simulink model "PSM_Commander_ATI"  (R2016a)
settings: Solver=ode3  StartTime=0.0  StopTime=inf  FixedStep=dt  RelTol=1e-3
InitFcn:
  | PSMCMD_DEPENDENCY
  | init_psm_cmd
  | init_scopes
  | init_udp
  | init_resolved_rates
  | ATI_Init_gamma
undefined symbols (not defined in the file or in its folder): A, ATI_torque_convert_to_Nmm, dt, epsilon_vec, f_bias, filter_coeffs_ATI, filter_coeffs_ATI_bias, H_organ2robot, H_robot2organ, inv_T, K_adm, N_ATI, N_ATI_bias, R_organ2robot, R_robot2organ, Rft2organ, scale_vec, v_limits
libraries: slrtlib x5, simulink x4, dspswit3 x4, xpcobsoletelib x3, xpcrtudplib x2, dspsigops x1
settings Model: Creator=Andrea  LastModifiedBy=Long
settings SolverCC: EnableConcurrentExecution=on
settings DataIOCC: LimitDataPoints=on  SaveFormat=Array  SignalLoggingSaveFormat=ModelDataLogs
settings OptimizationCC: BlockReduction=off  OptimizeBlockIOStorage=off  BufferReuse=off  GlobalBufferReuse=off  ExpressionFolding=off  ExpressionDepthLimit=2147483647  LocalBlockOutputs=off  OptimizeModelRefInitCode=on
settings DebuggingCC: UnderspecifiedInitializationDetection=Classic  MergeDetectMultiDrivingBlocksExec=none  SolverPrmCheckMsg=warning  MultiTaskCondExecSysMsg=warning  MultiTaskRateTransMsg=warning  FcnCallInpInsideContextMsg=UseLocalSettings  StateNameClashWarn=warning
settings HardwareCC: ProdBitPerPointer=32  ProdLargestAtomicFloat=None  ProdWordSize=32  ProdLongLongMode=on  ProdHWDeviceType=Generic->32-bit x86 compatible
settings ModelReferenceCC: PropagateSignalLabelsOutOfModel=off
settings SFSimCC: SimParseCustomCode=off
settings RTWCC: SystemTargetFile=slrtert.tlc  TemplateMakefile=slrtert_default_tmf  Description=Simulink Real-Time (ERT)  RTWCompilerOptimization=on
settings CodeAppCC: CustomSymbolStrType=$N$R$M  InternalIdentifier=Classic
settings SimulinkRealTimeERTCC: TargetFcnLib=ansi_tfl_table_tmw.mat  GenFloatMathFcnCalls=NOT IN USE  TargetLangStandard=C89/C90 (ANSI)  CodeReplacementLibrary=XPC_BLAS  UtilityFuncGeneration=Auto  ERTMultiwordTypeDef=System defined  ERTMultiwordLength=256  MultiwordLength=2048  GenerateFullHeader=on  InferredTypesCompatibility=off  GenerateSampleERTMain=off  GenerateTestInterfaces=off  ModelReferenceCompliant=on  ParMdlRefBuildCompliant=on  CompOptLevelCompliant=on  ConcurrentExecutionCompliant=on  IncludeMdlTerminateFcn=on  GeneratePreprocessorConditionals=Disable all  CombineOutputUpdateFcns=off  CombineSignalStateStructs=off  SuppressErrorStatus=off  ERTFirstTimeCompliant=off  IncludeFileDelimiter=Auto  ERTCustomFileBanners=off  SupportAbsoluteTime=on  LogVarNameModifier=rt_  MatFileLogging=on  MultiInstanceERTCode=off  CodeInterfacePackaging=Nonreusable function  SupportNonFinite=on  SupportComplex=on  PurelyIntegerCode=off  SupportContinuousTime=on  SupportNonInlinedSFcns=on  SupportVariableSizeSignals=off  ParenthesesLevel=Nominal  CastingMode=Nominal  MATLABClassNameForMDSCustomization=xpcAperiodicCustomization  ModelStepFunctionPrototypeControlCompliant=off  CPPClassGenCompliant=off  AutosarCompliant=off  GRTInterface=on  GenerateAllocFcn=off  UseToolchainInfoCompliant=off  GenerateSharedConstants=on  ExtModeTransport=0  ExtModeStaticAlloc=off  ExtModeStaticAllocSize=1000000  ExtModeTesting=off  InlinedParameterPlacement=Hierarchical  TargetOS=BareBoardExample  MultiInstanceErrorCode=Error  RateGroupingCode=on  RootIOFormat=Individual arguments  RTWCAPIRootIO=off  EnableDataOwnership=off  ERTFilePackagingFormat=Modular  PreserveExpressionOrder=off  PreserveIfCondition=off  ConvertIfToSwitch=off  PreserveExternInFcnDecls=on  SuppressUnreachableDefaultCases=off  EnableSignedLeftShifts=on  EnableSignedRightShifts=on  IndentStyle=K&R  IndentSize=2  EnableUserReplacementTypes=off  MaxIdInt32=MAX_int32_T  MinIdInt32=MIN_int32_T  MaxIdUint32=MAX_uint32_T  MaxIdInt16=MAX_int16_T  MinIdInt16=MIN_int16_T  MaxIdUint16=MAX_uint16_T  MaxIdInt8=MAX_int8_T  MinIdInt8=MIN_int8_T  MaxIdUint8=MAX_uint8_T  BooleanTrueId=true  BooleanFalseId=false  MemSecPackage=--- None ---  MemSecDataConstants=Default  MemSecDataIO=Default  MemSecDataInternal=Default  MemSecDataParameters=Default  MemSecFuncInitTerm=Default  MemSecFuncExecute=Default  MemSecFuncSharedUtil=Default  GlobalDataDefinition=Auto  GlobalDataReference=Auto  GenerateASAP2=off  ERTSrcFileBannerTemplate=ert_code_template.cgt  ERTHdrFileBannerTemplate=ert_code_template.cgt  ERTDataSrcFileTemplate=ert_code_template.cgt  ERTDataHdrFileTemplate=ert_code_template.cgt  ERTCustomFileTemplate=example_file_process.tlc  SignalDisplayLevel=10  ParamTuneLevel=10  InitialValueSource=Model  RTWCAPISignals=off  RTWCAPIParams=on  RTWCAPIStates=off  RL32ModeModifier=Real-Time  ExtMode=on  ExtModeMexFile=ext_xpc  ExtModeIntrfLevel=Level2 - Open  ExtModeArmWhenConnect=off  RL32LogTETModifier=on  RL32LogBufSizeModifier=100000  xPCTaskExecutionProfile=off  xPCRL32EventNumber=5000  RL32IRQSourceModifier=Timer  xPCIRQSourceBoard=None/Other  xPCIOIRQSlot=-1  xpcObjCom=off  xPCGenerateASAP2=off  xPCGenerateXML=off  RL32ObjectName=tg  xPCisDownloadable=off  xPCisDefaultEnv=on  xPCisModelTimeout=on  xPCModelTimeoutSecs=5  xpcDblBuff=off  xPCLoadParamSetFile=off  xPCConcurrentTasks=off  xPCEnableSFAnimation=off
settings ConfigComp: CovModelRefEnable=Off

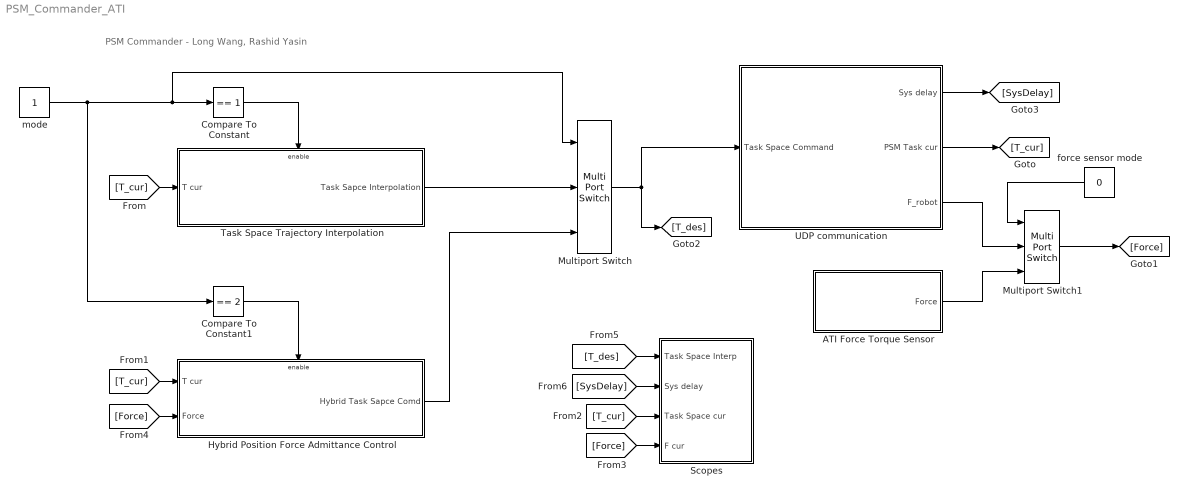
== system PSM_Commander_ATI ==
  note: PSM Commander - Long Wang, Rashid Yasin
  ATI Force Torque Sensor : Subsystem
  Compare To Constant : simulink/Logic and Bit Operations/Compare To Constant  relop===  const=1  OutDataTypeStr=boolean
  Compare To Constant1 : simulink/Logic and Bit Operations/Compare To Constant  relop===  const=2  OutDataTypeStr=boolean
  Hybrid Position Force Admittance Control : Subsystem  TreatAsAtomicUnit=on
  Multiport Switch : MultiPortSwitch  Inputs=2
  Multiport Switch1 : MultiPortSwitch  Inputs=2
  Scopes : Subsystem
  Task Space Trajectory Interpolation : Subsystem  TreatAsAtomicUnit=on
  UDP communication : Subsystem
  force sensor mode : Constant  Value=0
  mode : Constant
  wires:
  Compare To Constant/1 -> Task Space Trajectory Interpolation/Enable
  mode/1 -> Multiport Switch/1, Compare To Constant/1, Compare To Constant1/1
  Compare To Constant1/1 -> Hybrid Position Force Admittance Control/Enable
  Task Space Trajectory Interpolation/1(Task Sapce Interpolation) -> Multiport Switch/2
  Hybrid Position Force Admittance Control/1(Hybrid Task Sapce Comd) -> Multiport Switch/3
  UDP communication/2(PSM Task cur) -> [T_cur]
  [T_cur] -> Task Space Trajectory Interpolation/1(T cur)
  [T_cur] -> Hybrid Position Force Admittance Control/1(T cur)
  [T_cur] -> Scopes/3(Task Space cur)
  [Force] -> Scopes/4(F cur)
  [Force] -> Hybrid Position Force Admittance Control/2(Force)
  Multiport Switch/1 -> UDP communication/1(Task Space Command), [T_des]
  UDP communication/1(Sys delay) -> [SysDelay]
  UDP communication/3(F_robot) -> Multiport Switch1/2
  ATI Force Torque Sensor/1(Force) -> Multiport Switch1/3
  force sensor mode/1 -> Multiport Switch1/1
  Multiport Switch1/1 -> [Force]
  [T_des] -> Scopes/1("Task Space Interp ")
  [SysDelay] -> Scopes/2(Sys delay)

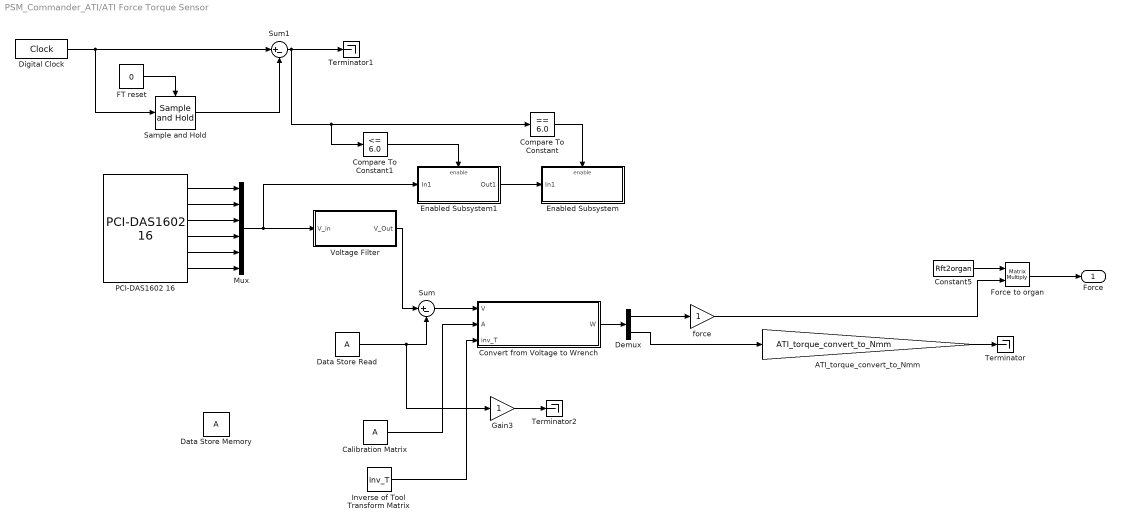
== system PSM_Commander_ATI/ATI Force Torque Sensor ==
  ATI_torque_convert_to_Nmm : Gain  Gain=ATI_torque_convert_to_Nmm
  Calibration Matrix : Constant  Value=A
  Compare To Constant : simulink/Logic and Bit Operations/Compare To Constant  relop===  const=6.0  OutDataTypeStr=uint8  ZeroCross=off
  Compare To Constant1 : simulink/Logic and Bit Operations/Compare To Constant  relop=<=  const=6.0  OutDataTypeStr=uint8  ZeroCross=off
  Constant5 : Constant  Value=Rft2organ
  "Convert from Voltage to Wrench " : MATLAB Function  TreatAsAtomicUnit=on
  Data Store Memory : DataStoreMemory  ReadBeforeWriteMsg=warning  WriteAfterWriteMsg=warning  WriteAfterReadMsg=warning  InitialValue=[0;0;0;0;0;0]  ShowAdditionalParam=off
  Data Store Read : DataStoreRead  SampleTime=0
  Demux : Demux  Outputs=2
  Digital Clock : DigitalClock  SampleTime=dt
  Enabled Subsystem : Subsystem  TreatAsAtomicUnit=on
  Enabled Subsystem1 : Subsystem  TreatAsAtomicUnit=on
  FT reset : Constant  Value=0
  Force to organ : Product  Multiplication=Matrix(*)
  Gain3 : Gain
  Inverse of Tool Transform Matrix : Constant  Value=inv_T  VectorParams1D=off
  Mux : Mux  Inputs=6
  "PCI-DAS1602 16 " : xpcobsoletelib/Measurement Computing obs/A//D/PCI-DAS1602 16   channel=6  range=+-10V  mux=Differential (8 channels)  sampletime=dt  slot=[5 4]
  Sample and Hold : dspsigops/Sample and Hold  trig=Rising edge  initCond=0  latchinput=off
  Sum : Sum  Inputs=|+-
  Sum1 : Sum  Inputs=|+-
  Terminator : Terminator
  Terminator1 : Terminator
  Terminator2 : Terminator
  Voltage Filter : Subsystem
  force : Gain
  Force : Outport
  wires:
  Mux/1 -> Voltage Filter/1(V_in), Enabled Subsystem1/1(In1)
  Calibration Matrix/1 -> "Convert from Voltage to Wrench "/2(A)
  Inverse of Tool Transform Matrix/1 -> "Convert from Voltage to Wrench "/3(inv_T)
  Sum/1 -> "Convert from Voltage to Wrench "/1(V)
  Voltage Filter/1(V_Out) -> Sum/1
  Data Store Read/1 -> Sum/2, Gain3/1
  Enabled Subsystem1/1(Out1) -> Enabled Subsystem/1(In1)
  Compare To Constant/1 -> Enabled Subsystem/Enable
  Gain3/1 -> Terminator2/1
  Compare To Constant1/1 -> Enabled Subsystem1/Enable
  "PCI-DAS1602 16 "/1 -> Mux/1
  "PCI-DAS1602 16 "/2 -> Mux/2
  "PCI-DAS1602 16 "/3 -> Mux/3
  "PCI-DAS1602 16 "/4 -> Mux/4
  "PCI-DAS1602 16 "/5 -> Mux/5
  "PCI-DAS1602 16 "/6 -> Mux/6
  Digital Clock/1 -> Sum1/1, Sample and Hold/1
  Sum1/1 -> Terminator1/1, Compare To Constant/1, Compare To Constant1/1
  Sample and Hold/1 -> Sum1/2
  FT reset/1 -> Sample and Hold/Trigger
  Demux/1 -> force/1
  Demux/2 -> ATI_torque_convert_to_Nmm/1
  ATI_torque_convert_to_Nmm/1 -> Terminator/1
  force/1 -> Force to organ/2
  Force to organ/1 -> Force/1
  "Convert from Voltage to Wrench "/1(W) -> Demux/1
  Constant5/1 -> Force to organ/1

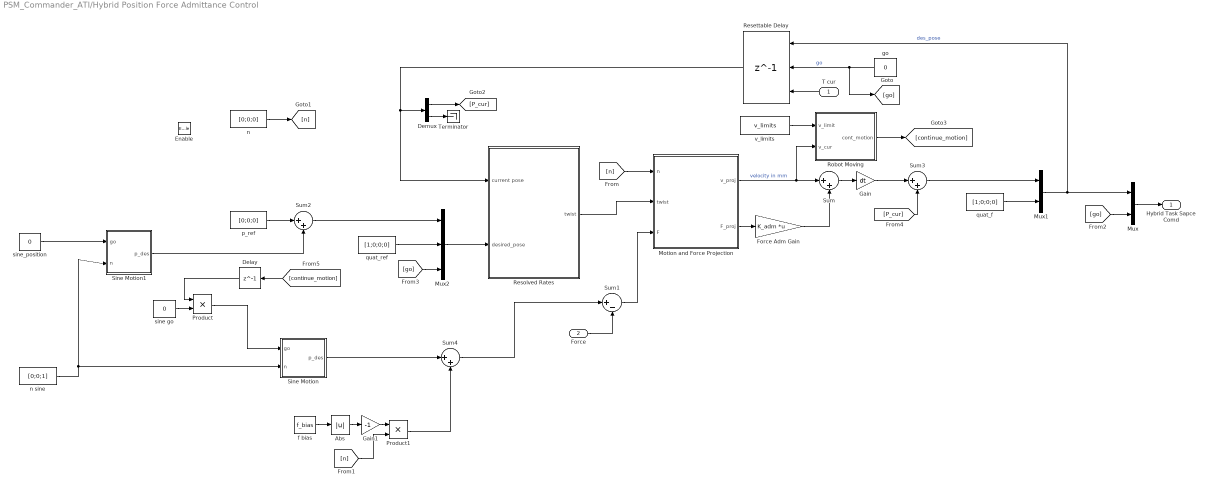
== system PSM_Commander_ATI/Hybrid Position Force Admittance Control ==
  T cur : Inport
  Force : Inport  Port=2
  Enable : EnablePort  StatesWhenEnabling=reset
  Abs : Abs
  Delay : Delay  DelayLength=1  InitialCondition=0
  Demux : Demux  Outputs=[3,4]
  Force Adm Gain : Gain  Gain=K_adm  Multiplication=Matrix(K*u)
  Gain : Gain  Gain=dt
  Gain1 : Gain  Gain=-1
  Motion and Force Projection : Subsystem
  Mux : Mux  Inputs=[7,1]
  Mux1 : Mux  Inputs=[3,4]
  Mux2 : Mux  Inputs=[3,4,1]
  Product : Product
  Product1 : Product
  Resettable Delay : Delay  DelayLength=1  InitialConditionSource=Input port  ExternalReset=Either  SampleTime=dt
      settings: InputPortMap=u0,r5,p4
  Resolved Rates : Subsystem
  Robot Moving : Subsystem  TreatAsAtomicUnit=on
  Sine Motion : Subsystem
  Sine Motion1 : Subsystem
  Sum{,2..4} (4 alike) : Sum  Inputs=|++
  Sum1 : Sum  Inputs=|+-
  Terminator : Terminator
  f bias : Constant  Value=f_bias
  go : Constant  Value=0
  n : Constant  Value=[0;0;0]
  n sine : Constant  Value=[0;0;1]
  p_ref : Constant  Value=[0;0;0]
  quat_f : Constant  Value=[1;0;0;0]
  quat_ref : Constant  Value=[1;0;0;0]
  sine go : Constant  Value=0
  sine_position : Constant  Value=0
  v_limits : Constant  Value=v_limits
  Hybrid Task Sapce Comd : Outport  InitialOutput=zeros(8,1)
  wires:
  [go] -> Mux/2
  go/1 -> [go], Resettable Delay/2  "go"
  Mux1/1 -> Mux/1, Resettable Delay/1  "des_pose"
  Mux/1 -> Hybrid Task Sapce Comd/1
  Resolved Rates/1(twist) -> Motion and Force Projection/2(twist)
  quat_ref/1 -> Mux2/2
  [go] -> Mux2/3
  Mux2/1 -> Resolved Rates/2(desired_pose)
  [n] -> Motion and Force Projection/1(n)
  Motion and Force Projection/2(F_proj) -> Force Adm Gain/1
  Motion and Force Projection/1(v_proj) -> Robot Moving/2(v_cur), Sum/1  "velocity in mm"
  Force Adm Gain/1 -> Sum/2
  Force/1 -> Sum1/2
  Sum1/1 -> Motion and Force Projection/3(F)
  p_ref/1 -> Sum2/1
  n/1 -> [n]
  n sine/1 -> Sine Motion1/2(n), Sine Motion/2(n)
  sine go/1 -> Product/2
  T cur/1 -> Resettable Delay/3
  Sine Motion/1(p_des) -> Sum4/1
  Sum2/1 -> Mux2/1
  quat_f/1 -> Mux1/2
  Sum/1 -> Gain/1
  Sum3/1 -> Mux1/1
  Demux/2 -> Terminator/1
  Resettable Delay/1 -> Resolved Rates/1(current pose), Demux/1
  Demux/1 -> [P_cur]
  [P_cur] -> Sum3/2
  Gain/1 -> Sum3/1
  Product/1 -> Sine Motion/1(go)
  Delay/1 -> Product/1
  Sum4/1 -> Sum1/1
  f bias/1 -> Abs/1
  [n] -> Product1/2
  Abs/1 -> Gain1/1
  Gain1/1 -> Product1/1
  Product1/1 -> Sum4/2
  sine_position/1 -> Sine Motion1/1(go)
  Sine Motion1/1(p_des) -> Sum2/2
  [continue_motion] -> Delay/1
  Robot Moving/1(cont_motion) -> [continue_motion]
  v_limits/1 -> Robot Moving/1(v_limit)

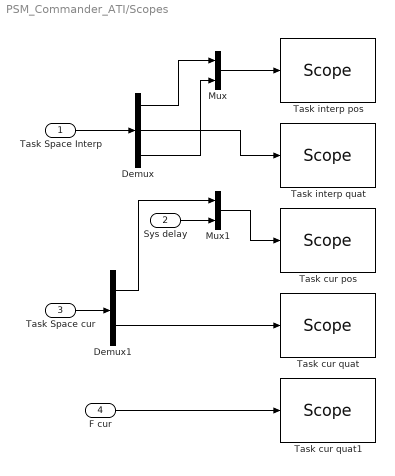
== system PSM_Commander_ATI/Scopes ==
  "Task Space Interp " : Inport
  Sys delay : Inport  Port=2
  Task Space cur : Inport  Port=3
  F cur : Inport  Port=4
  Demux : Demux  Outputs=[3,4,1]
  Demux1 : Demux  Outputs=[3,4]
  Mux : Mux  Inputs=2
  Mux1 : Mux  Inputs=2
  Task cur pos : slrtlib/Displays and Logging/Scope   scopeno=3  scopetype=Target  autostart=on  viewmode=Numerical  formatstr=Scope_format_Task_cur_p  grid=on  ylimits=[0,0]  nosamples=25  noprepostsamples=0  interleave=1  triggermode=FreeRun  triggersignal=1  trigsignalfromport=off  triggerlevel=0.0  triggerslope=Either  triggerscope=1  triggersample=0  filename=data.dat  mode=Lazy  writesize=512  autorestart=off  dynamicfilemode=off  maxwritefilesize=512*1024^2
  Task cur quat : slrtlib/Displays and Logging/Scope   scopeno=4  scopetype=Target  autostart=on  viewmode=Numerical  formatstr=Scope_format_Task_cur_quat  grid=on  ylimits=[0,0]  nosamples=25  noprepostsamples=0  interleave=1  triggermode=FreeRun  triggersignal=1  trigsignalfromport=off  triggerlevel=0.0  triggerslope=Either  triggerscope=1  triggersample=0  filename=data.dat  mode=Lazy  writesize=512  autorestart=off  dynamicfilemode=off  maxwritefilesize=512*1024^2
  Task cur quat1 : slrtlib/Displays and Logging/Scope   scopeno=5  scopetype=Target  autostart=on  viewmode=Numerical  formatstr=Scope_format_Task_cur_force  grid=on  ylimits=[0,0]  nosamples=25  noprepostsamples=0  interleave=1  triggermode=FreeRun  triggersignal=1  trigsignalfromport=off  triggerlevel=0.0  triggerslope=Either  triggerscope=1  triggersample=0  filename=data.dat  mode=Lazy  writesize=512  autorestart=off  dynamicfilemode=off  maxwritefilesize=512*1024^2
  "Task interp pos " : slrtlib/Displays and Logging/Scope   scopeno=1  scopetype=Target  autostart=on  viewmode=Numerical  formatstr=Scope_format_Task_interp_p  grid=on  ylimits=[0,0]  nosamples=25  noprepostsamples=0  interleave=1  triggermode=FreeRun  triggersignal=1  trigsignalfromport=off  triggerlevel=0.0  triggerslope=Either  triggerscope=1  triggersample=0  filename=data.dat  mode=Lazy  writesize=512  autorestart=off  dynamicfilemode=off  maxwritefilesize=512*1024^2
  Task interp quat : slrtlib/Displays and Logging/Scope   scopeno=2  scopetype=Target  autostart=on  viewmode=Numerical  formatstr=Scope_format_Task_interp_quat  grid=on  ylimits=[0,0]  nosamples=25  noprepostsamples=0  interleave=1  triggermode=FreeRun  triggersignal=1  trigsignalfromport=off  triggerlevel=0.0  triggerslope=Either  triggerscope=1  triggersample=0  filename=data.dat  mode=Lazy  writesize=512  autorestart=off  dynamicfilemode=off  maxwritefilesize=512*1024^2
  wires:
  "Task Space Interp "/1 -> Demux/1
  Demux/2 -> Task interp quat/1
  Demux/1 -> Mux/1
  Demux/3 -> Mux/2
  Mux/1 -> "Task interp pos "/1
  Task Space cur/1 -> Demux1/1
  Demux1/2 -> Task cur quat/1
  Demux1/1 -> Mux1/1
  Sys delay/1 -> Mux1/2
  Mux1/1 -> Task cur pos/1
  F cur/1 -> Task cur quat1/1

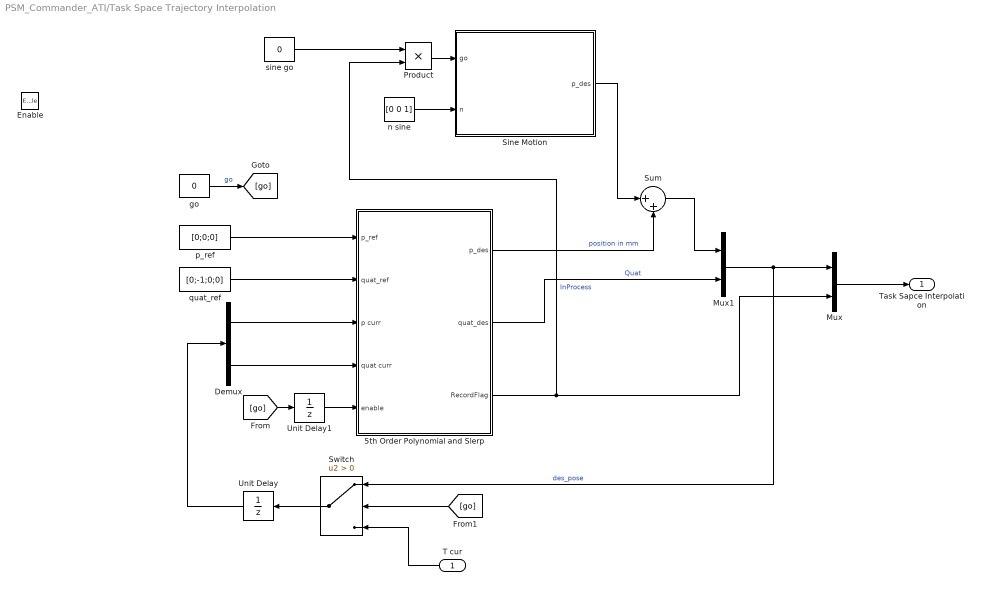
== system PSM_Commander_ATI/Task Space Trajectory Interpolation ==
  T cur : Inport
  Enable : EnablePort  StatesWhenEnabling=reset
  5th Order Polynomial and Slerp : Subsystem
  Demux : Demux  Outputs=[3,4]
  Mux : Mux  Inputs=[7,1]
  Mux1 : Mux  Inputs=[3,4]
  Product : Product
  Sine Motion : Subsystem
  Sum : Sum  Inputs=|++
  Switch : Switch  Criteria=u2 > Threshold
  Unit Delay : UnitDelay  InitialCondition=[zeros(3,1);[1;0;0;0]]  SampleTime=-1
  Unit Delay1 : UnitDelay  SampleTime=-1
  go : Constant  Value=0
  n sine : Constant  Value=[0 0 1]
  p_ref : Constant  Value=[0;0;0]
  quat_ref : Constant  Value=[0;-1;0;0]
  sine go : Constant  Value=0
  Task Sapce Interpolation : Outport  InitialOutput=zeros(8,1)
  wires:
  p_ref/1 -> 5th Order Polynomial and Slerp/1(p_ref)
  quat_ref/1 -> 5th Order Polynomial and Slerp/2(quat_ref)
  5th Order Polynomial and Slerp/3(RecordFlag) -> Product/2, Mux/2  "InProcess"
  Mux/1 -> Task Sapce Interpolation/1
  5th Order Polynomial and Slerp/2(quat_des) -> Mux1/2  "Quat"
  Mux1/1 -> Switch/1, Mux/1  "des_pose"
  go/1 -> [go]  "go"
  [go] -> Unit Delay1/1
  T cur/1 -> Switch/3
  [go] -> Switch/2
  Switch/1 -> Unit Delay/1
  Demux/1 -> 5th Order Polynomial and Slerp/3(p curr)
  Demux/2 -> 5th Order Polynomial and Slerp/4(quat curr)
  Unit Delay1/1 -> 5th Order Polynomial and Slerp/5(enable)
  Unit Delay/1 -> Demux/1
  n sine/1 -> Sine Motion/2(n)
  Sine Motion/1(p_des) -> Sum/1
  5th Order Polynomial and Slerp/1(p_des) -> Sum/2  "position in mm"
  Sum/1 -> Mux1/1
  Product/1 -> Sine Motion/1(go)
  sine go/1 -> Product/1

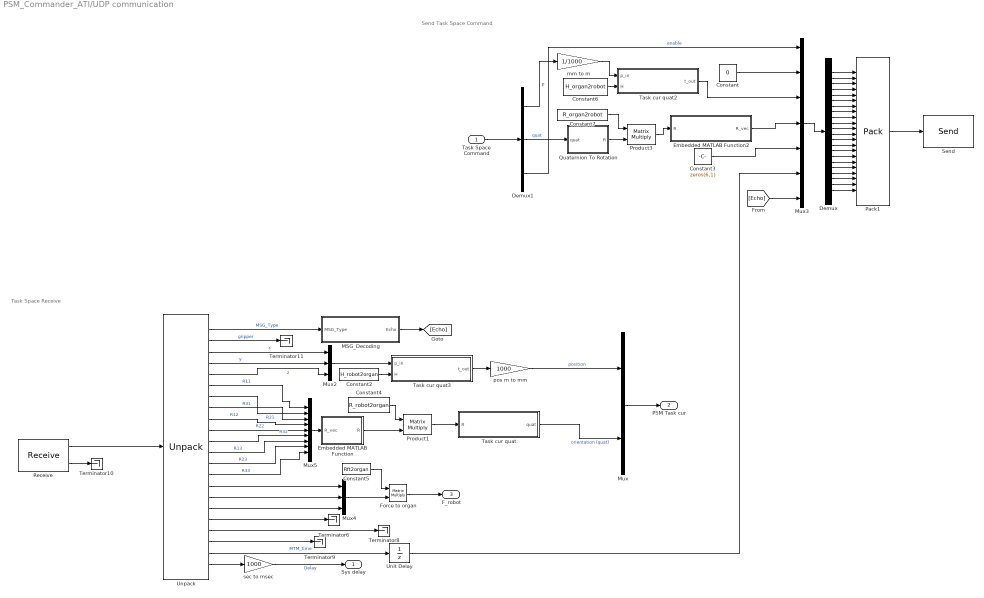
== system PSM_Commander_ATI/UDP communication ==
  note: Task Space Receive
  note: Send Task Space Command
  Task Space Command : Inport
  Constant : Constant  Value=0
  Constant2 : Constant  Value=H_robot2organ
  Constant3 : Constant  Value=zeros(6,1)
  Constant4 : Constant  Value=R_robot2organ
  Constant5 : Constant  Value=Rft2organ
  Constant6 : Constant  Value=H_organ2robot
  Constant7 : Constant  Value=R_organ2robot
  Demux : Demux  Outputs=22
  Demux1 : Demux  Outputs=[3,4,1]
  Embedded MATLAB Function : MATLAB Function  TreatAsAtomicUnit=on
  Embedded MATLAB Function2 : MATLAB Function  TreatAsAtomicUnit=on
  Force to organ : Product  Multiplication=Matrix(*)
  MSG_Decoding : MATLAB Function  TreatAsAtomicUnit=on
  Mux : Mux  Inputs=[3,4]
  Mux2 : Mux  Inputs=3
  Mux3 : Mux  Inputs=7
  Mux4 : Mux  Inputs=3
  Mux5 : Mux  Inputs=9
  Pack1 : xpcobsoletelib/Utilities/Pack   datatypes={'double' 'double' 'double' 'double' 'double' 'double' 'double' 'double' 'double' 'double' 'double' 'double' 'double' 'double' 'double' 'double' 'double' 'double' 'double' 'double' 'double' 'double'}  byteAlign=1
  Product1 : Product  Multiplication=Matrix(*)
  Product3 : Product  Multiplication=Matrix(*)
  Quaternion To Rotation : MATLAB Function  TreatAsAtomicUnit=on
  "Receive " : xpcrtudplib/Legacy UDP/Receive   ipAddress=0.0.0.0  ipPort=10006  width=22*8  vblLen=off  sampletime=dt_udp
  "Send " : xpcrtudplib/Legacy UDP/Send   ipAddress=192.168.1.11  ipPort=10005  localPort=-1  vblLen=off  sampletime=dt_udp
  Task cur quat : MATLAB Function  TreatAsAtomicUnit=on
  Task cur quat2 : MATLAB Function  TreatAsAtomicUnit=on
  Task cur quat3 : MATLAB Function  TreatAsAtomicUnit=on
  Terminator{6,8..11} (5 alike) : Terminator
  Unit Delay : UnitDelay  SampleTime=-1
  Unpack : xpcobsoletelib/Utilities/Unpack   dimensions={1,1,1,1,1,1,1,1,1,1,1,1,1,1,1,1,1,1,1,1,1,1}  datatypes={'double' 'double' 'double' 'double' 'double' 'double' 'double' 'double' 'double' 'double' 'double' 'double' 'double' 'double' 'double' 'double' 'double' 'double' 'double' 'double' 'double' 'double'}  byteAlign=1
  mm to m : Gain  Gain=1/1000
  pos m to mm : Gain  Gain=1000
  sec to msec : Gain  Gain=1000
  Sys delay : Outport
  PSM Task cur : Outport  Port=2
  F_robot : Outport  Port=3
  wires:
  Task Space Command/1 -> Demux1/1
  Mux/1 -> PSM Task cur/1
  Unpack/19 -> Terminator8/1
  Unpack/20 -> Terminator9/1
  Unpack/18 -> Terminator6/1
  Unpack/17 -> Mux4/3
  Unpack/16 -> Mux4/2
  Unpack/15 -> Mux4/1
  Mux5/1 -> Embedded MATLAB Function/1(R_vec)
  Unpack/14 -> Mux5/9  "R33"
  Unpack/13 -> Mux5/8  "R23"
  Unpack/12 -> Mux5/7  "R13"
  Unpack/11 -> Mux5/6  "R32"
  Unpack/10 -> Mux5/5  "R22"
  Unpack/9 -> Mux5/4  "R12"
  Unpack/8 -> Mux5/3  "R31"
  Unpack/7 -> Mux5/2  "R21"
  Unpack/6 -> Mux5/1  "R11"
  Unpack/22 -> sec to msec/1
  Mux2/1 -> Task cur quat3/1(p_in)
  Unpack/3 -> Mux2/1  "x"
  Unpack/4 -> Mux2/2  "y"
  Unpack/5 -> Mux2/3  "z"
  "Receive "/1 -> Unpack/1
  Unpack/1 -> MSG_Decoding/1(MSG_Type)  "MSG_Type"
  Unpack/2 -> Terminator11/1  "gripper"
  pos m to mm/1 -> Mux/1  "position"
  Unpack/21 -> Unit Delay/1  "MTM_time"
  "Receive "/2 -> Terminator10/1
  Task cur quat/1(quat) -> Mux/2  "orientation (quat)"
  Pack1/1 -> "Send "/1
  Mux3/1 -> Demux/1
  Demux/1 -> Pack1/1
  Demux/2 -> Pack1/2
  Demux/3 -> Pack1/3
  Demux/4 -> Pack1/4
  Demux/5 -> Pack1/5
  Demux/6 -> Pack1/6
  Demux/7 -> Pack1/7
  Demux/8 -> Pack1/8
  Demux/9 -> Pack1/9
  Demux/10 -> Pack1/10
  Demux/11 -> Pack1/11
  Demux/12 -> Pack1/12
  Demux/13 -> Pack1/13
  Demux/14 -> Pack1/14
  Demux/15 -> Pack1/15
  Demux/16 -> Pack1/16
  Demux/17 -> Pack1/17
  Demux/18 -> Pack1/18
  Demux/19 -> Pack1/19
  Demux/20 -> Pack1/20
  Demux/21 -> Pack1/21
  Demux1/2 -> Quaternion To Rotation/1(quat)  "quat"
  Quaternion To Rotation/1(R) -> Product3/2
  MSG_Decoding/1(Echo) -> [Echo]
  [Echo] -> Mux3/7
  Constant/1 -> Mux3/2
  Demux1/1 -> mm to m/1  "p"
  Embedded MATLAB Function2/1(R_vec) -> Mux3/4
  Unit Delay/1 -> Mux3/6
  Constant3/1 -> Mux3/5
  Task cur quat2/1(t_out) -> Mux3/3
  sec to msec/1 -> Sys delay/1  "Delay"
  Demux1/3 -> Mux3/1  "enable"
  Demux/22 -> Pack1/22
  Mux4/1 -> Force to organ/2
  mm to m/1 -> Task cur quat2/1(p_in)
  Constant2/1 -> Task cur quat3/2(H)
  Constant4/1 -> Product1/1
  Embedded MATLAB Function/1(R) -> Product1/2
  Constant5/1 -> Force to organ/1
  Force to organ/1 -> F_robot/1
  Product3/1 -> Embedded MATLAB Function2/1(R)
  Constant6/1 -> Task cur quat2/2(H)
  Constant7/1 -> Product3/1
  Task cur quat3/1(t_out) -> pos m to mm/1
  Product1/1 -> Task cur quat/1(R)

== system PSM_Commander_ATI/ATI Force Torque Sensor/Enabled Subsystem ==
  In1 : Inport
  Enable : EnablePort
  Data Store Write : DataStoreWrite
  wires:
  In1/1 -> Data Store Write/1

== system PSM_Commander_ATI/ATI Force Torque Sensor/Enabled Subsystem1 ==
  In1 : Inport
  Enable : EnablePort
  Voltage Filter Bias : Subsystem
  Out1 : Outport
  wires:
  In1/1 -> Voltage Filter Bias/1(V_in)
  Voltage Filter Bias/1(V_Out) -> Out1/1

== system PSM_Commander_ATI/ATI Force Torque Sensor/Voltage Filter ==
  V_in : Inport
  Discrete FIR Filter : DiscreteFir  CoefSource=Input port  AccumDataTypeStr=Inherit: Same as product output
      settings: InputPortMap=u0,u1
  Gain : Gain  Gain=1/N_ATI
  filter_coeffs : Constant  Value=filter_coeffs_ATI
  V_Out : Outport
  wires:
  V_in/1 -> Discrete FIR Filter/1
  Discrete FIR Filter/1 -> Gain/1
  filter_coeffs/1 -> Discrete FIR Filter/2
  Gain/1 -> V_Out/1

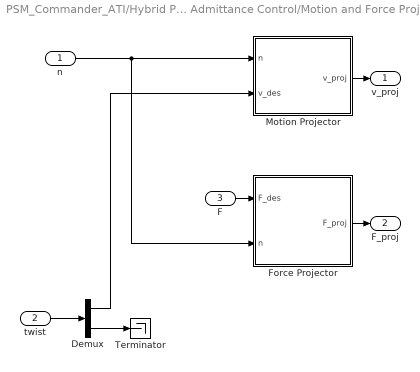
== system PSM_Commander_ATI/Hybrid Position Force Admittance Control/Motion and Force Projection ==
  n : Inport
  twist : Inport  Port=2
  F : Inport  Port=3
  Demux : Demux  Outputs=[3,3]
  Force Projector : Subsystem  TreatAsAtomicUnit=on
  Motion Projector : Subsystem  TreatAsAtomicUnit=on
  Terminator : Terminator
  v_proj : Outport
  F_proj : Outport  Port=2
  wires:
  F/1 -> Force Projector/1(F_des)
  Force Projector/1(F_proj) -> F_proj/1
  Motion Projector/1(v_proj) -> v_proj/1
  n/1 -> Force Projector/2(n), Motion Projector/1(n)
  twist/1 -> Demux/1
  Demux/1 -> Motion Projector/2(v_des)
  Demux/2 -> Terminator/1

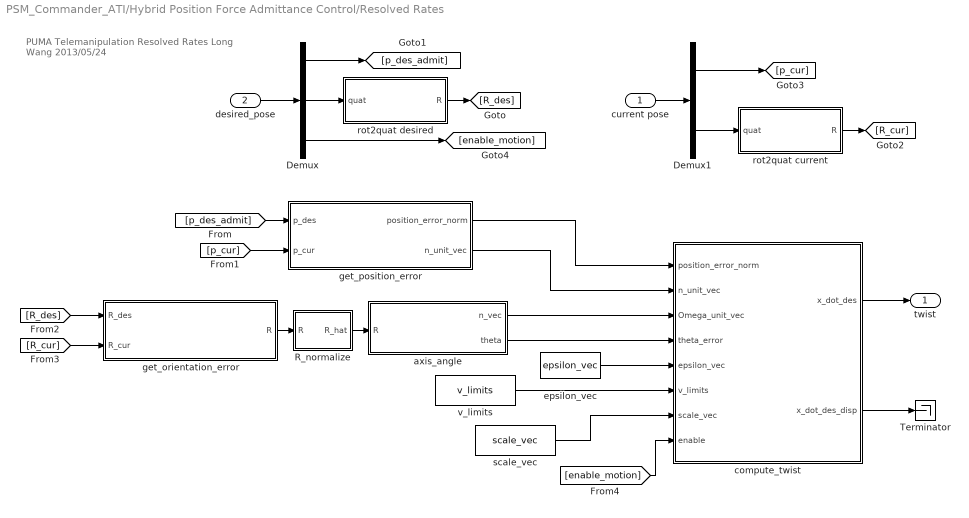
== system PSM_Commander_ATI/Hybrid Position Force Admittance Control/Resolved Rates ==
  note: PUMA Telemanipulation Resolved Rates
      | Long Wang
      | 2013/05/24
  current pose : Inport
  desired_pose : Inport  Port=2
  Demux : Demux  Outputs=[3,4,1]
  Demux1 : Demux  Outputs=[3,4]
  R_normalize : MATLAB Function  TreatAsAtomicUnit=on
  Terminator : Terminator
  axis_angle : MATLAB Function  TreatAsAtomicUnit=on
  compute_twist : MATLAB Function  TreatAsAtomicUnit=on
  epsilon_vec : Constant  Value=epsilon_vec
  get_orientation_error : MATLAB Function  TreatAsAtomicUnit=on
  get_position_error : MATLAB Function  TreatAsAtomicUnit=on
  rot2quat current : MATLAB Function  TreatAsAtomicUnit=on
  rot2quat desired : MATLAB Function  TreatAsAtomicUnit=on
  scale_vec : Constant  Value=scale_vec
  v_limits : Constant  Value=v_limits
  twist : Outport
  wires:
  current pose/1 -> Demux1/1
  get_position_error/1(position_error_norm) -> compute_twist/1(position_error_norm)
  get_position_error/2(n_unit_vec) -> compute_twist/2(n_unit_vec)
  v_limits/1 -> compute_twist/6(v_limits)
  epsilon_vec/1 -> compute_twist/5(epsilon_vec)
  Demux1/1 -> [p_cur]
  compute_twist/1(x_dot_des) -> twist/1
  scale_vec/1 -> compute_twist/7(scale_vec)
  get_orientation_error/1(R) -> R_normalize/1(R)
  [p_des_admit] -> get_position_error/1(p_des)
  [p_cur] -> get_position_error/2(p_cur)
  [R_des] -> get_orientation_error/1(R_des)
  [R_cur] -> get_orientation_error/2(R_cur)
  [enable_motion] -> compute_twist/8(enable)
  axis_angle/1(n_vec) -> compute_twist/3(Omega_unit_vec)
  axis_angle/2(theta) -> compute_twist/4(theta_error)
  R_normalize/1(R_hat) -> axis_angle/1(R)
  compute_twist/2(x_dot_des_disp) -> Terminator/1
  desired_pose/1 -> Demux/1
  Demux/3 -> [enable_motion]
  Demux/1 -> [p_des_admit]
  Demux/2 -> rot2quat desired/1(quat)
  rot2quat desired/1(R) -> [R_des]
  rot2quat current/1(R) -> [R_cur]
  Demux1/2 -> rot2quat current/1(quat)

== system PSM_Commander_ATI/Hybrid Position Force Admittance Control/Robot Moving ==
  v_limit : Inport
  v_cur : Inport  Port=2
  endMotion : MATLAB Function  TreatAsAtomicUnit=on
  cont_motion : Outport
  wires:
  v_limit/1 -> endMotion/2(v_limits)
  endMotion/1(y) -> cont_motion/1
  v_cur/1 -> endMotion/1(v_cur)

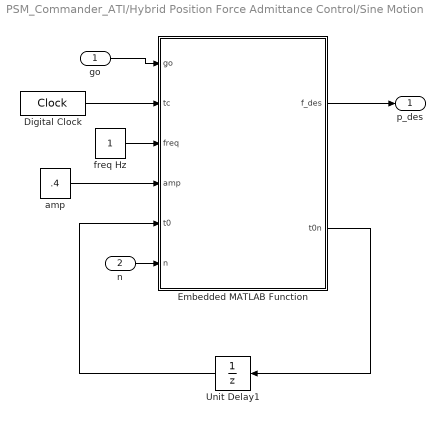
== system PSM_Commander_ATI/Hybrid Position Force Admittance Control/Sine Motion ==
  go : Inport
  n : Inport  Port=2
  Digital Clock : DigitalClock  SampleTime=dt
  Embedded MATLAB Function : MATLAB Function  TreatAsAtomicUnit=on
  Unit Delay1 : UnitDelay  SampleTime=dt
  amp : Constant  Value=.4  SampleTime=dt
  freq Hz : Constant  SampleTime=dt
  p_des : Outport
  wires:
  Digital Clock/1 -> Embedded MATLAB Function/2(tc)
  freq Hz/1 -> Embedded MATLAB Function/3(freq)
  Embedded MATLAB Function/2(t0n) -> Unit Delay1/1
  Unit Delay1/1 -> Embedded MATLAB Function/5(t0)
  amp/1 -> Embedded MATLAB Function/4(amp)
  Embedded MATLAB Function/1(f_des) -> p_des/1
  go/1 -> Embedded MATLAB Function/1(go)
  n/1 -> Embedded MATLAB Function/6(n)

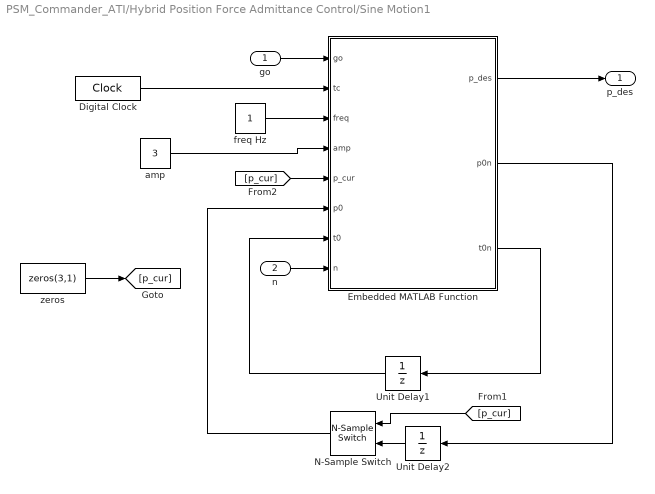
== system PSM_Commander_ATI/Hybrid Position Force Admittance Control/Sine Motion1 ==
  go : Inport
  n : Inport  Port=2
  Digital Clock : DigitalClock  SampleTime=dt
  Embedded MATLAB Function : MATLAB Function  TreatAsAtomicUnit=on
  N-Sample Switch : dspswit3/N-Sample Switch  N=1  reset=off  TriggerType=Rising edge  Ts=dt
  Unit Delay1 : UnitDelay  SampleTime=dt
  Unit Delay2 : UnitDelay  SampleTime=dt
  amp : Constant  Value=3  SampleTime=dt
  freq Hz : Constant  SampleTime=dt
  zeros : Constant  Value=zeros(3,1)  SampleTime=dt
  p_des : Outport
  wires:
  zeros/1 -> [p_cur]
  n/1 -> Embedded MATLAB Function/8(n)
  go/1 -> Embedded MATLAB Function/1(go)
  [p_cur] -> Embedded MATLAB Function/5(p_cur)
  Embedded MATLAB Function/1(p_des) -> p_des/1
  Embedded MATLAB Function/2(p0n) -> Unit Delay2/1
  amp/1 -> Embedded MATLAB Function/4(amp)
  Unit Delay1/1 -> Embedded MATLAB Function/7(t0)
  Embedded MATLAB Function/3(t0n) -> Unit Delay1/1
  freq Hz/1 -> Embedded MATLAB Function/3(freq)
  Digital Clock/1 -> Embedded MATLAB Function/2(tc)
  [p_cur] -> N-Sample Switch/1
  Unit Delay2/1 -> N-Sample Switch/2
  N-Sample Switch/1 -> Embedded MATLAB Function/6(p0)

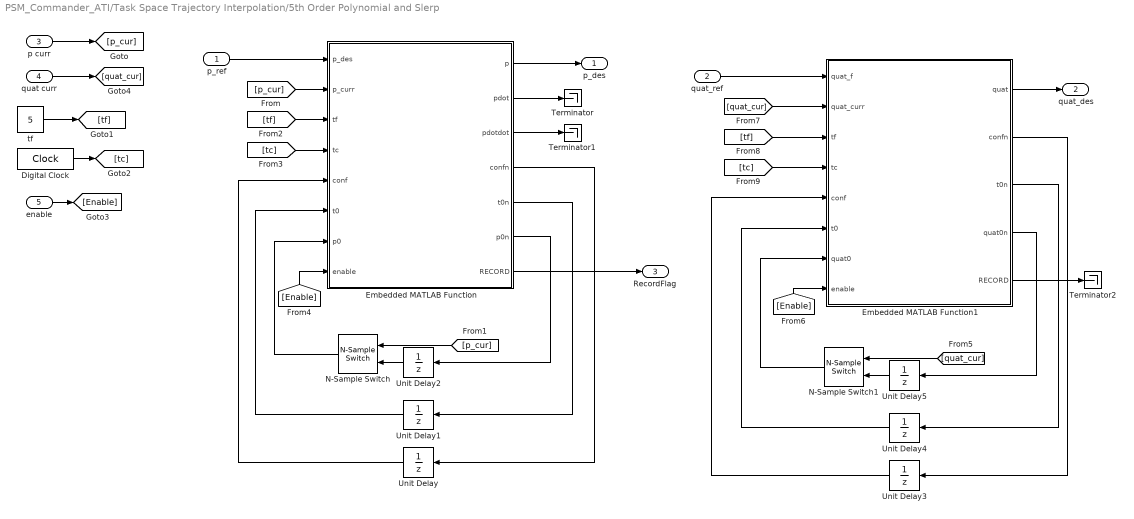
== system PSM_Commander_ATI/Task Space Trajectory Interpolation/5th Order Polynomial and Slerp ==
  p_ref : Inport
  quat_ref : Inport  Port=2
  p curr : Inport  Port=3
  quat curr : Inport  Port=4
  enable : Inport  Port=5
  Digital Clock : DigitalClock  SampleTime=dt
  Embedded MATLAB Function : MATLAB Function  TreatAsAtomicUnit=on
  Embedded MATLAB Function1 : MATLAB Function  TreatAsAtomicUnit=on
  N-Sample Switch : dspswit3/N-Sample Switch  N=1  reset=off  TriggerType=Rising edge  Ts=dt
  N-Sample Switch1 : dspswit3/N-Sample Switch  N=1  reset=off  TriggerType=Rising edge  Ts=dt
  Terminator : Terminator
  Terminator1 : Terminator
  Terminator2 : Terminator
  Unit Delay{,1..4} (5 alike) : UnitDelay  SampleTime=dt
  Unit Delay5 : UnitDelay  InitialCondition=[1;0;0;0]  SampleTime=dt
  tf : Constant  Value=5  SampleTime=dt
  p_des : Outport
  quat_des : Outport  Port=2
  RecordFlag : Outport  Port=3
  wires:
  Embedded MATLAB Function/4(confn) -> Unit Delay/1
  Unit Delay/1 -> Embedded MATLAB Function/5(conf)
  Embedded MATLAB Function/5(t0n) -> Unit Delay1/1
  Embedded MATLAB Function/6(p0n) -> Unit Delay2/1
  Unit Delay1/1 -> Embedded MATLAB Function/6(t0)
  p_ref/1 -> Embedded MATLAB Function/1(p_des)
  Embedded MATLAB Function/2(pdot) -> Terminator/1
  Embedded MATLAB Function/3(pdotdot) -> Terminator1/1
  N-Sample Switch/1 -> Embedded MATLAB Function/7(p0)
  Unit Delay2/1 -> N-Sample Switch/2
  p curr/1 -> [p_cur]
  [p_cur] -> Embedded MATLAB Function/2(p_curr)
  [p_cur] -> N-Sample Switch/1
  Embedded MATLAB Function/7(RECORD) -> RecordFlag/1
  Embedded MATLAB Function/1(p) -> p_des/1
  tf/1 -> [tf]
  Digital Clock/1 -> [tc]
  [tf] -> Embedded MATLAB Function/3(tf)
  [tc] -> Embedded MATLAB Function/4(tc)
  enable/1 -> [Enable]
  [Enable] -> Embedded MATLAB Function/8(enable)
  quat_ref/1 -> Embedded MATLAB Function1/1(quat_f)
  quat curr/1 -> [quat_cur]
  Embedded MATLAB Function1/3(t0n) -> Unit Delay4/1
  Embedded MATLAB Function1/4(quat0n) -> Unit Delay5/1
  Unit Delay4/1 -> Embedded MATLAB Function1/6(t0)
  N-Sample Switch1/1 -> Embedded MATLAB Function1/7(quat0)
  Unit Delay5/1 -> N-Sample Switch1/2
  [quat_cur] -> N-Sample Switch1/1
  Embedded MATLAB Function1/2(confn) -> Unit Delay3/1
  Unit Delay3/1 -> Embedded MATLAB Function1/5(conf)
  [Enable] -> Embedded MATLAB Function1/8(enable)
  [quat_cur] -> Embedded MATLAB Function1/2(quat_curr)
  [tf] -> Embedded MATLAB Function1/3(tf)
  [tc] -> Embedded MATLAB Function1/4(tc)
  Embedded MATLAB Function1/1(quat) -> quat_des/1
  Embedded MATLAB Function1/5(RECORD) -> Terminator2/1

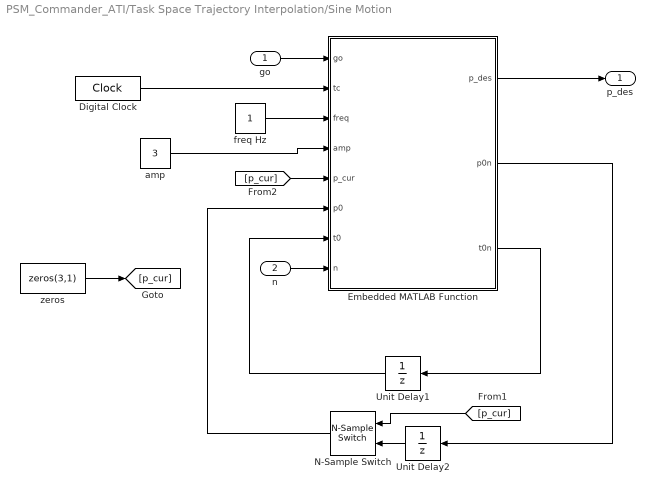
== system PSM_Commander_ATI/Task Space Trajectory Interpolation/Sine Motion ==
  go : Inport
  n : Inport  Port=2
  Digital Clock : DigitalClock  SampleTime=dt
  Embedded MATLAB Function : MATLAB Function  TreatAsAtomicUnit=on
  N-Sample Switch : dspswit3/N-Sample Switch  N=1  reset=off  TriggerType=Rising edge  Ts=dt
  Unit Delay1 : UnitDelay  SampleTime=dt
  Unit Delay2 : UnitDelay  SampleTime=dt
  amp : Constant  Value=3  SampleTime=dt
  freq Hz : Constant  SampleTime=dt
  zeros : Constant  Value=zeros(3,1)  SampleTime=dt
  p_des : Outport
  wires:
  N-Sample Switch/1 -> Embedded MATLAB Function/6(p0)
  Unit Delay2/1 -> N-Sample Switch/2
  [p_cur] -> N-Sample Switch/1
  Digital Clock/1 -> Embedded MATLAB Function/2(tc)
  freq Hz/1 -> Embedded MATLAB Function/3(freq)
  Embedded MATLAB Function/3(t0n) -> Unit Delay1/1
  Unit Delay1/1 -> Embedded MATLAB Function/7(t0)
  amp/1 -> Embedded MATLAB Function/4(amp)
  Embedded MATLAB Function/2(p0n) -> Unit Delay2/1
  Embedded MATLAB Function/1(p_des) -> p_des/1
  [p_cur] -> Embedded MATLAB Function/5(p_cur)
  go/1 -> Embedded MATLAB Function/1(go)
  n/1 -> Embedded MATLAB Function/8(n)
  zeros/1 -> [p_cur]

== system PSM_Commander_ATI/ATI Force Torque Sensor/Enabled Subsystem1/Voltage Filter Bias ==
  V_in : Inport
  Discrete FIR Filter : DiscreteFir  CoefSource=Input port  AccumDataTypeStr=Inherit: Same as product output
      settings: InputPortMap=u0,u1
  Gain : Gain  Gain=1/N_ATI_bias
  filter_coeffs : Constant  Value=filter_coeffs_ATI_bias
  V_Out : Outport
  wires:
  Gain/1 -> V_Out/1
  filter_coeffs/1 -> Discrete FIR Filter/2
  Discrete FIR Filter/1 -> Gain/1
  V_in/1 -> Discrete FIR Filter/1

== system PSM_Commander_ATI/Hybrid Position Force Admittance Control/Motion and Force Projection/Force Projector ==
  F_des : Inport
  n : Inport  Port=2
  Projector : MATLAB Function  TreatAsAtomicUnit=on
  F_proj : Outport
  wires:
  Projector/1(y) -> F_proj/1
  F_des/1 -> Projector/1(F)
  n/1 -> Projector/2(N)

== system PSM_Commander_ATI/Hybrid Position Force Admittance Control/Motion and Force Projection/Motion Projector ==
  n : Inport
  v_des : Inport  Port=2
  Projector : MATLAB Function  TreatAsAtomicUnit=on
  v_proj : Outport
  wires:
  n/1 -> Projector/2(N)
  Projector/1(y) -> v_proj/1
  v_des/1 -> Projector/1(F)

== matlab function PSM_Commander_ATI/Hybrid Position Force Admittance Control/Resolved Rates/rot2quat current ==
  data: quat input; R output
function R = rotation2quat(quat)
%#codegen
R=quat2rot(quat);

== matlab function PSM_Commander_ATI/Hybrid Position Force Admittance Control/Resolved Rates/rot2quat desired ==
  data: quat input; R output
function R = rotation2quat(quat)
%#codegen
R=quat2rot(quat);

== matlab function PSM_Commander_ATI/Task Space Trajectory Interpolation/Sine Motion/Embedded MATLAB Function ==
  data: p_des output; p0n output; go input; tc input; freq input; amp input; p_cur input; p0 input; t0 input; t0n output; n input
function [p_des,p0n,t0n] = fcn(go,tc,freq,amp,p_cur,p0,t0,n)
%#eml
if go
    t = tc - t0;
    p_des = p0 + amp*sin(2*pi*freq*t)*n;
    t0n = t0;
    p0n = p0;
else
    p_des = p_cur;
    p0n = p_cur;
    t0n = tc;
end

== matlab function PSM_Commander_ATI/Hybrid Position Force Admittance Control/Robot Moving/endMotion ==
  data: v_cur input; v_limits input; y output
function y = fcn(v_cur,v_limits)
vmin=v_limits(1,1);

y =norm(v_cur)>vmin*.5;

== matlab function PSM_Commander_ATI/Hybrid Position Force Admittance Control/Sine Motion/Embedded MATLAB Function ==
  data: f_des output; go input; tc input; freq input; amp input; t0 input; t0n output; n input
function [f_des,t0n] = cos_force(go,tc,freq,amp,t0,n)
%#eml
if go
    t = tc - t0;
    f_des = (amp*cos(2*pi*freq*t)-amp)*n;
    t0n = t0;
else
    f_des = 0*n;
    t0n = tc;
end

== matlab function PSM_Commander_ATI/Hybrid Position Force Admittance Control/Sine Motion1/Embedded MATLAB Function ==
  data: p_des output; p0n output; go input; tc input; freq input; amp input; p_cur input; p0 input; t0 input; t0n output; n input
function [p_des,p0n,t0n] = fcn(go,tc,freq,amp,p_cur,p0,t0,n)
%#eml
if go
    t = tc - t0;
    p_des = p0 + amp*sin(2*pi*freq*t)*n;
    t0n = t0;
    p0n = p0;
else
    p_des = p_cur;
    p0n = p_cur;
    t0n = tc;
end

== matlab function PSM_Commander_ATI/Hybrid Position Force Admittance Control/Motion and Force Projection/Motion Projector/Projector ==
  data: F input; N input; y output
function y = fcn(F,N)

Omega_f = N * N';
Omega_m = eye(3) - Omega_f;

y = Omega_m * F;

== matlab function PSM_Commander_ATI/Hybrid Position Force Admittance Control/Motion and Force Projection/Force Projector/Projector ==
  data: F input; N input; y output
function y = fcn(F,N)

Omega_f = N * N';

y = Omega_f * F;

== matlab function PSM_Commander_ATI/Hybrid Position Force Admittance Control/Resolved Rates/axis_angle ==
  data: R input; n_vec output; theta output
function [n_vec, theta] = get_axis_angle(R)
%#codegen
% Jason Pile
%axis_angle(R) gives the rotation axis and the rotation angle extracted
%from rotation matrix R
%   n_vec=unit vector along rotation axis
%   theta=rotation angle about rotation axis
    theta=acos(1/2*(trace(R)-1));
    if abs(theta)<(10^-4)
        n_vec=[1;0;0];
    elseif abs(theta-pi)<(10^-4)
        n_vec=[-1;0;0];        
    else
        n_cross=1/(2*sin(theta))*(R-R');
        n_vec=[-n_cross(2,3);n_cross(1,3);-n_cross(1,2)];
        n_vec=n_vec/norm(n_vec);
    end
end

== matlab function PSM_Commander_ATI/UDP communication/Task cur quat2 ==
  data: p_in input; t_out output; H input
function t_out   = pos_Transform(p_in,H)
   t_full = H*[p_in;1];
   t_out=t_full(1:3);
end

== matlab function PSM_Commander_ATI/Hybrid Position Force Admittance Control/Resolved Rates/get_position_error ==
  data: p_des input; p_cur input; position_error_norm output; n_unit_vec output
%#codegen
function [position_error_norm,n_unit_vec] = GetPositionErr(p_des,p_cur)
% Long Wang 2013/06/02
p_des = p_des(:); % make sure column vector
p_cur = p_cur(:);
position_error_vec = p_des-p_cur;
position_error_norm = norm(position_error_vec);
%% compute linear velocity direction
if position_error_norm==0
    n_unit_vec = [1;0;0];
else
    n_unit_vec = position_error_vec/position_error_norm;
end

== matlab function PSM_Commander_ATI/UDP communication/Task cur quat3 ==
  data: p_in input; t_out output; H input
function t_out   = pos_Transform(p_in,H)
   t_full = H*[p_in;1];
   t_out=t_full(1:3);
end

== matlab function PSM_Commander_ATI/ATI Force Torque Sensor/Convert from Voltage to Wrench  ==
  data: V input; W output; A input; inv_T input
function W = Convert_Function(V,A,inv_T)%A_vec,p)

W = inv_T*A*V;

== matlab function PSM_Commander_ATI/Hybrid Position Force Admittance Control/Resolved Rates/get_orientation_error ==
  data: R_des input; R_cur input; R output
%#codegen
function R  = GetOrientationErr(R_des,R_cur)
% Long Wang
% 2013/06/02
% orientation error R_des=R*R_cur is a rotayionn sequence in world frame
R = R_des * (R_cur');

== matlab function PSM_Commander_ATI/Hybrid Position Force Admittance Control/Resolved Rates/R_normalize ==
  data: R input; R_hat output
function R_hat = R_norm(R)
%#codegen
rx = R(:,1);
rx = rx/norm(rx);
ry = R(:,2);
ry = ry/norm(ry);
rz = cross(rx,ry);
rz = rz/norm(rz);
R_hat = [rx,ry,rz];
end

== matlab function PSM_Commander_ATI/Hybrid Position Force Admittance Control/Resolved Rates/compute_twist ==
  data: position_error_norm input; n_unit_vec input; Omega_unit_vec input; theta_error input; epsilon_vec input; v_limits input; scale_vec input; x_dot_des output; enable input; x_dot_des_disp output
%#codegen

function [x_dot_des,x_dot_des_disp]= compute_twist(position_error_norm,n_unit_vec, Omega_unit_vec, theta_error,epsilon_vec,v_limits,scale_vec,enable)
%% compute_twist :
%   Description:    This embedded matlab function computes the desired twist
%                   of the end-effector to follow a straight line through p_curr
%                   and p_des and bring the R_curr to R_des using angle/axis
%                   representation
%
%   References:     Siciliano, Sciavicco, Villani, Oriolo, Robotics: Modelling, Planning and Control
%                   1. angle/axis pg 52
%                   2. trajectories pg 161
%
%                   Nabil's notes on Resolved Rate Algorithm
%
%   Inputs:         1. p_des is the desired end effector position
%                   2. R_des is the desired end effectror orientation
%                   3. p_curr is the current position of the robot's operational point
%                   5. R_curr is the current orientation of the robot's tool
%   Outputs:        1. x_des is the desired twist of the robot end-effector
%                   2. theta is the orientation error (to be removed in final version)
%--------------------------------------------------------------------------
if enable == 1  % if motion is enabled
    Vmin = v_limits(1,1); % [m/s]
    Vmax = v_limits(2,1); % [m/s]
    OmegaMin = v_limits(3,1);   %rad/s
    OmegaMax = v_limits(4,1);   %rad/s
    
    position_epsilon=epsilon_vec(1);
    orientation_epsilon=epsilon_vec(2);

    
    %%  check for convergence
%     lin_vel_ratio=Vmax/Vmin;
    lin_vel_ratio = scale_vec(1,1);
    ang_vel_ratio=OmegaMax/OmegaMin;
    %     if abs(position_error) < position_epsilon && abs(theta_error) < orientation_epsilon
    %         x_dot_des = zeros(6,1);
    %         %%if not converged calculate target speed
    %
    %     else
    
    if abs(position_error_norm)>position_epsilon*lin_vel_ratio;
%         alpha_translation_t=1; 
        LinVelMag = Vmax; %go at maximal speed
    elseif abs(position_error_norm)<position_epsilon;
%         alpha_translation_t=0;
        LinVelMag = 0;
    else
        alpha_translation_t=...
            (position_error_norm - position_epsilon)/...
            (lin_vel_ratio*position_epsilon - position_epsilon);
        LinVelMag = (Vmax - Vmin)*alpha_translation_t + Vmin;
%         safety check
        if (LinVelMag >Vmax) 
            LinVelMag =Vmax;
        end
    end
    
       
    
    
    if abs(theta_error)>orientation_epsilon*ang_vel_ratio
        alpha_rotation_t=1; %go at maximal speed
    elseif abs(theta_error)<orientation_epsilon,
        alpha_rotation_t=0;
    else
        alpha_rotation_t=theta_error/(ang_vel_ratio*orientation_epsilon);
    end
    
    AngVelMag=alpha_rotation_t*OmegaMax;
    
    % compute desired twist
    x_dot_des = [LinVelMag*n_unit_vec
        AngVelMag*Omega_unit_vec];
    % end
else  %enable=0
    x_dot_des = zeros(6,1);
end
    x_dot_des_disp = x_dot_des;
% safety by Long Wang
if (sum(isnan(x_dot_des))~=0)
    x_dot_des = zeros(6,1);
end

== matlab function PSM_Commander_ATI/Task Space Trajectory Interpolation/5th Order Polynomial and Slerp/Embedded MATLAB Function ==
  data: p output; p_des input; p_curr input; tf input; tc input; pdot output; pdotdot output; conf input; confn output; t0 input; t0n output; p0n output; p0 input; enable input; RECORD output
function [p,pdot,pdotdot,confn,t0n,p0n,RECORD] = fifth_order_p(p_des,p_curr,tf,tc,conf,t0,p0,enable)

n = 3;
RECORD = 0;

if enable == 0                  % Configuration space is not used (pdot = 0). 
    p = p_curr;
    pdotdot = zeros(n,1);
    pdot = zeros(n,1);          % However we do want to record the current 
    confn = 0;                  % position in order to be ready as soon 
    t0n = tc;                   % as the enable becomes 1. 
    p0n = p_curr;
else
    if (p_des-p0)'*(p_des-p0) > 0
        if conf == 0                % conf = 0 means that the 5th order poly 
            p0n = p0;               % is not configured for the desired trajectory.
            t0n = tc;               % Therefore, the block is initialized.
            confn = 1;
            pdot = zeros(n,1);
            p = p0;
            pdotdot = zeros(n,1);
        else
            p0n = p0;
            t0n = t0;
            confn = conf;
            % 5th order polynomial
            a0 = p0;
            a4 = -15*(p_des-p0);
            a3 = -2/3 * a4;
            a5 = -2/5 * a4;
            t = tc-t0;
            tau = t/tf;
            if t < tf
                RECORD = 1;
                p = a0 + a3 * tau^3 + a4 * tau^4 + a5 * tau^5;
                pdot = 3*a3*t^2/tf^3 + 4*a4*t^3/tf^4 + 5*a5*t^4/tf^5;
                pdotdot = 6*a3*t/tf^3 + 12*a4*t^2/tf^4 + 20*a5*t^3/tf^5;
            else
                p = p_des;
                pdot = zeros(n,1);
                pdotdot = zeros(n,1);
                p0n = p_des;
            end
        end
    else
        p = p_des;
        pdot = zeros(n,1);
        pdotdot = zeros(n,1);
        confn = 0;
        p0n = p0;
        t0n = t0;
    end
end
%------------------------------------------------------------------------

== matlab function PSM_Commander_ATI/UDP communication/MSG_Decoding ==
  data: MSG_Type input; Echo output
function Echo = Decode(MSG_Type)
%#codegen
% decode the message_type
% MSG_Type def
% bit0 = valid massage or not(enable or not)
% bit1 = time stamping requested or not (if should send back the local time or not)
enable = bitand(uint8(floor(MSG_Type)),2);
Echo= double(enable);

== matlab function PSM_Commander_ATI/UDP communication/Quaternion To Rotation ==
  data: quat input; R output
function R = fcn(quat)
%#eml
if norm(quat)==0
    quat = [1;0;0;0];
end
R = quat2rot(quat);

== matlab function PSM_Commander_ATI/UDP communication/Embedded MATLAB Function2 ==
  data: R input; R_vec output
function R_vec = R_to_vec(R)
%#eml
%%  This func will cast a [3x3] rotation matrix to [9x1]
%%  The mapping will be column matrix, see for yourself.
R_vec = R(:);

== matlab function PSM_Commander_ATI/Task Space Trajectory Interpolation/5th Order Polynomial and Slerp/Embedded MATLAB Function1 ==
  data: quat output; quat_f input; quat_curr input; tf input; tc input; conf input; confn output; t0 input; t0n output; quat0n output; quat0 input; enable input; RECORD output
function [quat,confn,t0n,quat0n,RECORD] = quat_slerp(quat_f,quat_curr,tf,tc,conf,t0,quat0,enable)
%%  modified version of 5th order poly for Slerp
%   
RECORD = 0;
if enable == 0                  % Configuration space is not used (pdot = 0). 
    quat = quat_curr;
    confn = 0;                  % position in order to be ready as soon 
    t0n = tc;                   % as the enable becomes 1. 
    quat0n = quat_curr;
else
    if (quat0'*quat_f)<1
        if conf == 0                % conf = 0 means that the 5th order poly 
            quat0n = quat0;               % is not configured for the desired trajectory.
            t0n = tc;               % Therefore, the block is initialized.
            confn = 1;
            quat = quat0;
        else
            quat0n = quat0;
            t0n = t0;
            confn = conf;
            % Slerp
            t = tc-t0;
            tau = t/tf;
            if t < tf
                RECORD = 1;
                quat = slerp(quat0,quat_f,tau);
            else
                quat = quat_f;
                quat0n = quat_f;
            end
        end
    else
        quat = quat_f;
        confn = 0;
        quat0n = quat0;
        t0n = t0;
    end
end
%------------------------------------------------------------------------

== matlab function PSM_Commander_ATI/UDP communication/Embedded MATLAB Function ==
  data: R_vec input; R output
function R = parse_rot(R_vec)
%#codegen
if norm(R_vec)==0
    R = eye(3);
else
    R = reshape(R_vec,3,3);
end

== matlab function PSM_Commander_ATI/UDP communication/Task cur quat ==
  data: R input; quat output
function quat   = convert_rot_to_quat(R)
   quat = rot2quat(R);
end
